simulink model "problem8"  (R2021a)
settings: Solver=VariableStepAuto  StartTime=0.0  StopTime=0.1  RelTol=1e-3
undefined symbols (not defined in the file): f1, f2, f3, f4, J, k, n, Tau1, Tau2, Tau3, Tau4, u1, u2, u3, u4
settings Model: Creator=Marti  LastModifiedBy=Marti

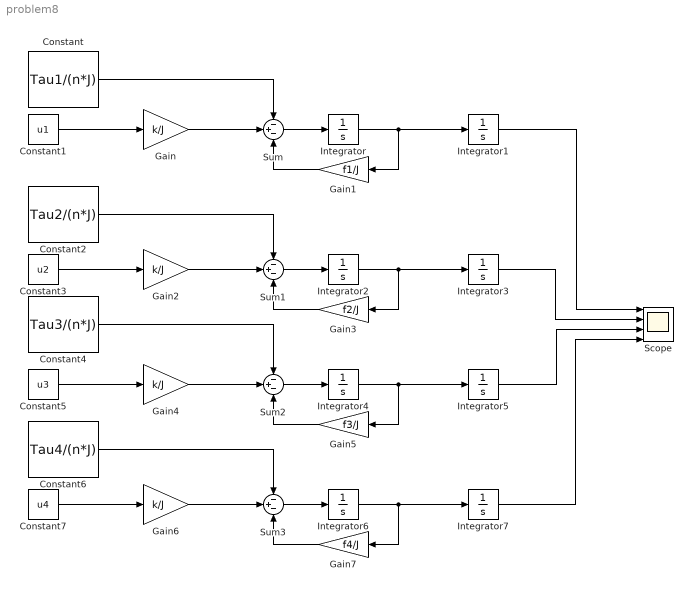
== system problem8 ==
  Constant : Constant  Value=Tau1/(n*J)
  Constant1 : Constant  Value=u1
  Constant2 : Constant  Value=Tau2/(n*J)
  Constant3 : Constant  Value=u2
  Constant4 : Constant  Value=Tau3/(n*J)
  Constant5 : Constant  Value=u3
  Constant6 : Constant  Value=Tau4/(n*J)
  Constant7 : Constant  Value=u4
  Gain{,2,4,6} (4 alike) : Gain  Gain=k/J
  Gain1 : Gain  Gain=f1/J
  Gain3 : Gain  Gain=f2/J
  Gain5 : Gain  Gain=f3/J
  Gain7 : Gain  Gain=f4/J
  Integrator{,1..7} (8 alike) : Integrator
  Scope : Scope  NumInputPorts=4
  Sum{,1..3} (4 alike) : Sum  Inputs=-+-
  wires:
  Gain/1 -> Sum/2
  Constant1/1 -> Gain/1
  Constant/1 -> Sum/1
  Integrator/1 -> Gain1/1, Integrator1/1
  Sum/1 -> Integrator/1
  Integrator1/1 -> Scope/1
  Gain1/1 -> Sum/3
  Constant2/1 -> Sum1/1
  Gain3/1 -> Sum1/3
  Integrator2/1 -> Gain3/1, Integrator3/1
  Sum1/1 -> Integrator2/1
  Constant3/1 -> Gain2/1
  Integrator3/1 -> Scope/2
  Constant5/1 -> Gain4/1
  Sum2/1 -> Integrator4/1
  Integrator4/1 -> Integrator5/1, Gain5/1
  Gain5/1 -> Sum2/3
  Constant4/1 -> Sum2/1
  Gain4/1 -> Sum2/2
  Gain6/1 -> Sum3/2
  Constant6/1 -> Sum3/1
  Gain7/1 -> Sum3/3
  Integrator6/1 -> Gain7/1, Integrator7/1
  Sum3/1 -> Integrator6/1
  Constant7/1 -> Gain6/1
  Integrator5/1 -> Scope/3
  Integrator7/1 -> Scope/4
  Gain2/1 -> Sum1/2
